simulink model "Open_Loop"  (Simulink 7.5)
settings: Solver=ode15s  StartTime=0.0  StopTime=4  RelTol=1e-3
libraries: powerlib x16, powerlib_extras x2, simulink x1
settings Model: Creator=lm  LastModifiedBy=lm

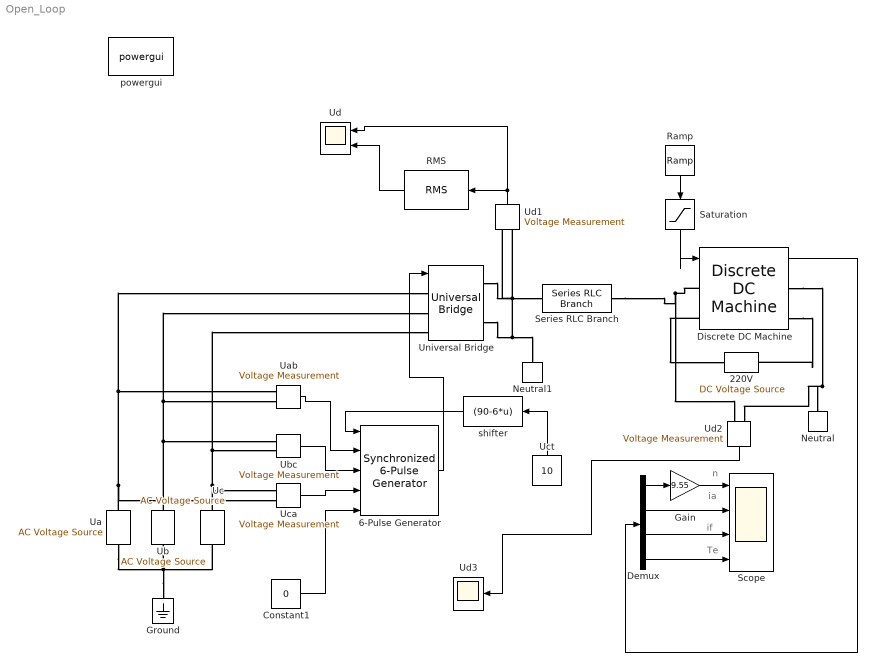
== system Open_Loop ==
  note: n
  note: ia
  note: if
  note: Te
  220V : powerlib/Electrical Sources/DC Voltage Source  DialogController=POWERSYS.PowerSysDialog  SystemSampleTime=-1  Amplitude=220  Measurements=None
  6-Pulse Generator : powerlib_extras/Control  Blocks/Synchronized 6-Pulse Generator  DialogController=POWERSYS.PowerSysDialog  SystemSampleTime=-1  freq=50  pwidth=5  Double_Pulse=on
  Constant1 : Constant  Value=0  OutDataType=fixdt(1, 16)  OutScaling=2^0
  Demux : Demux
  Discrete DC Machine : powerlib/Machines/Discrete DC Machine  DialogController=POWERSYS.PowerSysDialog  SystemSampleTime=-1  PresetModel=No  MechanicalLoad=Torque TL  FieldType=Wound  ShowDetailedParameters=on  RLa="[ 0.21  0.000021]"  RLf=[146.7 0]  Laf=0.84  MachineConstant=Torque constant (N.m/A)  Ke=1.8  Kt=1.8  J=0.57  Bm=0  Tf=0  w0=0  Ifinit=1  TsPowergui=0  TsBlock=-1
      settings: AttributesFormatString=\n
  Gain : Gain  Gain=9.55  ParameterDataType=fixdt(1, 16)  ParameterScaling=2^0  OutDataType=fixdt(1, 16)  OutScaling=2^0
  Ground : powerlib/Elements/Ground  DialogController=POWERSYS.PowerSysDialog  PhysicalDomain=powersysdomain  SubClassName=unknown  LeftPortType=p1  RightPortType=p1  LConnTagsString=a
  Neutral : powerlib/Elements/Neutral  DialogController=POWERSYS.PowerSysDialog  PhysicalDomain=powersysdomain  SubClassName=unknown  LeftPortType=p1  RightPortType=p1  LConnTagsString=a  NodeNumber=10
  Neutral1 : powerlib/Elements/Neutral  DialogController=POWERSYS.PowerSysDialog  PhysicalDomain=powersysdomain  SubClassName=unknown  LeftPortType=p1  RightPortType=p1  LConnTagsString=a  NodeNumber=10
  RMS : powerlib_extras/Measurements/RMS  DialogController=POWERSYS.PowerSysDialog  SystemSampleTime=-1  f1=60
  Ramp : simulink/Sources/Ramp  SystemSampleTime=-1  slope=100000  start=2.5  X0=0
  Saturation : Saturate  UpperLimit=22  LowerLimit=-171.45  LinearizeAsGain=off  OutDataType=fixdt(1, 16)  OutScaling=2^0
  Scope : Scope  NumInputPorts=4
      settings: YMin=1972.25~-0.025~1.42468~-0.025  YMax=1975~0.2~1.57464~0.275
  Series RLC Branch : powerlib/Elements/Series RLC Branch  DialogController=POWERSYS.PowerSysDialog  PhysicalDomain=powersysdomain  SubClassName=unknown  LeftPortType=p1  RightPortType=p1  LConnTagsString=__new0  RConnTagsString=__new0  BranchType=L  Resistance=1  Inductance=0.2  SetiL0=off  InitialCurrent=0  Capacitance=1e-6  Setx0=off  InitialVoltage=0  Measurements=None
  Ua : powerlib/Electrical Sources/AC Voltage Source  DialogController=POWERSYS.PowerSysDialog  SystemSampleTime=-1  Amplitude=123*sqrt(2)  Phase=0  Frequency=50  SampleTime=0  Measurements=None
  Uab : powerlib/Measurements/Voltage Measurement  DialogController=POWERSYS.PowerSysDialog  SystemSampleTime=-1  PhasorSimulation=off  OutputType=Complex  PSBequivalent=0
  Ub : powerlib/Electrical Sources/AC Voltage Source  DialogController=POWERSYS.PowerSysDialog  SystemSampleTime=-1  Amplitude=123*sqrt(2)  Phase=-120  Frequency=50  SampleTime=0  Measurements=None
  Ubc : powerlib/Measurements/Voltage Measurement  DialogController=POWERSYS.PowerSysDialog  SystemSampleTime=-1  PhasorSimulation=off  OutputType=Complex  PSBequivalent=0
  Uc : powerlib/Electrical Sources/AC Voltage Source  DialogController=POWERSYS.PowerSysDialog  SystemSampleTime=-1  Amplitude=123*sqrt(2)  Phase=-240  Frequency=50  SampleTime=0  Measurements=None
  Uca : powerlib/Measurements/Voltage Measurement  DialogController=POWERSYS.PowerSysDialog  SystemSampleTime=-1  PhasorSimulation=off  OutputType=Complex  PSBequivalent=0
  Uct : Constant  Value=10  OutDataType=fixdt(1, 16)  OutScaling=2^0
  Ud : Scope  NumInputPorts=2
      settings: YMin=-80~1.7e-005  YMax=0~2.125e-005
  Ud1 : powerlib/Measurements/Voltage Measurement  DialogController=POWERSYS.PowerSysDialog  SystemSampleTime=-1  PhasorSimulation=off  OutputType=Complex  PSBequivalent=0
  Ud2 : powerlib/Measurements/Voltage Measurement  DialogController=POWERSYS.PowerSysDialog  SystemSampleTime=-1  PhasorSimulation=off  OutputType=Complex  PSBequivalent=0
  Ud3 : Scope
      settings: TimeRange=4  SaveName=ScopeData2
  Universal Bridge : powerlib/Power Electronics/Universal Bridge  DialogController=POWERSYS.PowerSysDialog  SystemSampleTime=-1  Arms=3  SnubberResistance=1e6  SnubberCapacitance=inf  Device=Thyristors  Ron=1.3  Lon=0  ForwardVoltages="[  0  0  ]"  ForwardVoltage=0  GTOparameters=[ 10e-6 , 20e-6 ]  IGBTparameters=[ 1e-6 , 2e-6 ]  Measurements=Device voltages  Measurements_2=None  converterType=Rectifier
  powergui : powerlib/powergui  Priority=1  SystemSampleTime=-1  SimulationMode=Discrete  SampleTime=50e-6  frequency=60  SPID=off  DisableSnubberDevices=off  DisableRonSwitches=off  DisableVfSwitches=off  SwTol=0  Interpol=off  frequencyindice=0  echomessages=off  HookPort=off  DisplayEquations=off  FunctionMessages=off  EnableUseOfTLC=off  x0status=blocks  RestoreLinks=warning  ResistiveCurrentMeasurement=off  Ylog=off  Xlog=on  ShowGrid=off  save=off  variable=ZData  ZoomFFT=off  StartTime=0.0  cycles=1  DisplayStyle=1  FreqAxis=off  MaxFrequency=1000  frequencyindicesteady=1  display=off  methode=off
  shifter : Fcn  Expr=(90-6*u)
  wires:
  Constant1/1 -> 6-Pulse Generator/5
  Uca/1 -> 6-Pulse Generator/4
  Ubc/1 -> 6-Pulse Generator/3
  Uab/1 -> 6-Pulse Generator/2
  Uct/1 -> shifter/1
  shifter/1 -> 6-Pulse Generator/1
  Ramp/1 -> Saturation/1
  Saturation/1 -> Discrete DC Machine/1
  Discrete DC Machine/1 -> Demux/1
  Demux/2 -> Scope/2
  Demux/3 -> Scope/3
  Demux/4 -> Scope/4
  Demux/1 -> Gain/1
  Gain/1 -> Scope/1
  Ud1/1 -> RMS/1, Ud/1
  RMS/1 -> Ud/2
  Ud2/1 -> Ud3/1
  6-Pulse Generator/1 -> Universal Bridge/1
  connections:
  Ground/LConn1 -- Ua/LConn1 -- Ub/LConn1 -- Uc/LConn1
  Ua/RConn1 -- Universal Bridge/LConn1 -- Uab/LConn1 -- Uca/LConn2
  Ub/RConn1 -- Universal Bridge/LConn2 -- Uab/LConn2 -- Ubc/LConn1
  Uc/RConn1 -- Universal Bridge/LConn3 -- Ubc/LConn2 -- Uca/LConn1
  Universal Bridge/RConn1 -- Series RLC Branch/LConn1 -- Ud1/LConn1
  Universal Bridge/RConn2 -- Ud1/LConn2 -- Neutral1/LConn1
  Discrete DC Machine/LConn2 -- 220V/RConn1
  Discrete DC Machine/RConn2 -- 220V/LConn1
  Series RLC Branch/RConn1 -- Discrete DC Machine/LConn1 -- Ud2/LConn1
  Discrete DC Machine/RConn1 -- Ud2/LConn2 -- Neutral/LConn1
